simulink model "MODELO_CORRECTO_BERGMAN_BASE"  (R2019b)
settings: Solver=VariableStepAuto  StartTime=0.0  StopTime=50000  RelTol=1e-3
undefined symbols (not defined in the file): Gb, Ib, n, p1, p2, p3, p5, p6
libraries: simulink x29
settings Model: Creator=USUARIO  LastModifiedBy=USUARIO

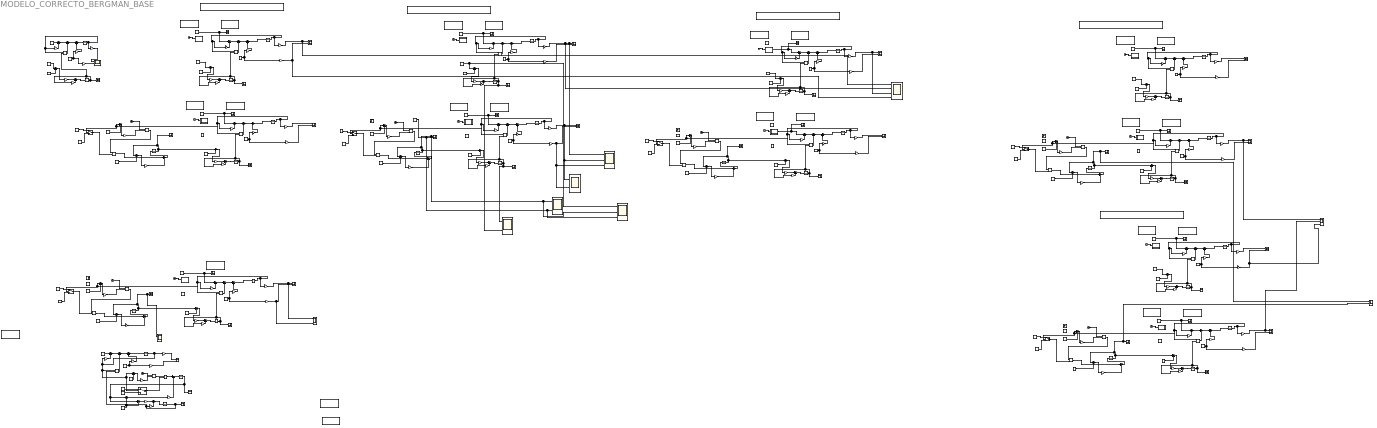
== system MODELO_CORRECTO_BERGMAN_BASE ==
  "    " : Gain  Gain=p6
  Clock{,1..17} (18 alike) : Clock
  Constant{1..11} (11 alike) : Constant  Value=0
  Factor conversión : Gain  Gain=18
  "Factor conversión    " : Gain  Gain=18
  Factor de conversión : Gain  Gain=18
  "Factor de conversión " : Gain  Gain=18
  False : Constant
  Gain{1,5,8,10,13..14,20,23,25..26,32,35,37..38,44,47,49..50,56,59,61,65,67,69,71,75} (26 alike) : Gain  Gain=p1
  Gain{2,11,15,17,27,29,39,41,51,53,62,68,70} (13 alike) : Gain  Gain=p3
  Gain{3..4,7,12,16,18..19,22,28,30..31,34,40,42..43,46,52,54..55,58,63..64} (22 alike) : Gain  Gain=18
  Gain{6,9,21,24,33,36,45,48,57,60,66,72,76} (13 alike) : Gain  Gain=p2
  "Glucosa " : Constant  Value=12
  Glucosa {2..5} (4 alike) : Constant  Value=7
  Glucosa basal : Constant  Value=Gb
  "Glucosa basal         " : Constant  Value=Gb
  Glucosa basal{1..4,9..10,13,17..18,21} (10 alike) : Constant  Value=4.5
  Glucosa basal{5,7,11,15,19,22} (6 alike) : Constant
  Glucosa basal{6,8,12,16,20,23} (6 alike) : Constant  Value=0
  Glucosa basal14 : Constant  Value=5.11
  Grafica ingesta D{1..10,12} (11 alike) : Scope
  Grafica ingesta D11 : Scope  NumInputPorts=2
  Gráfica de la glucosa : Scope  NumInputPorts=2
  Gráfica glucosa : Scope  NumInputPorts=2
  Gráfica insulina activa : Scope
  "Gráfica insulina activa       " : Scope
  Gráfica insulina variable : Scope
  INSULINA : Scope  NumInputPorts=2
  INSULINA{1..5} (5 alike) : Scope
  INSULINA7 : Scope  NumInputPorts=2
  Ib{,1..2,4..5} (5 alike) : Constant  Value=12
  Ib3 : Constant  Value=11
  Ingesta : Constant  Value=0
  "Ingesta      " : Constant  Value=0
  Ingesta 75 g1 : MATLAB Function  TreatAsAtomicUnit=on
  Ingesta 75 g10 : MATLAB Function  TreatAsAtomicUnit=on
  Ingesta 75 g11 : MATLAB Function  TreatAsAtomicUnit=on
  Ingesta 75 g2 : MATLAB Function  TreatAsAtomicUnit=on
  Ingesta 75 g3 : MATLAB Function  TreatAsAtomicUnit=on
  Ingesta 75 g4 : MATLAB Function  TreatAsAtomicUnit=on
  Ingesta 75 g5 : MATLAB Function  TreatAsAtomicUnit=on
  Ingesta 75 g6 : MATLAB Function  TreatAsAtomicUnit=on
  Ingesta 75 g7 : MATLAB Function  TreatAsAtomicUnit=on
  Ingesta 75 g8 : MATLAB Function  TreatAsAtomicUnit=on
  Ingesta 75 g9 : MATLAB Function  TreatAsAtomicUnit=on
  "Insulina basal     " : Constant  Value=Ib
  Insulina basal{1..6,8..11} (10 alike) : Constant  Value=12
  Insulina basal7 : Constant  Value=11
  Insulina constante : Constant  Value=Ib
  Integrator{1,5,16,19,21,24} (6 alike) : Integrator  InitialCondition=7.5
  Integrator{3,8,10,13,32} (5 alike) : Integrator  InitialCondition=4.5
  Integrator{4,11,14,17,22,27,30} (7 alike) : Integrator  InitialCondition=12
  Integrator{2,6..7,9,12,15,18,20,23,25,28,31,33} (13 alike) : Integrator
  Integrator26 : Integrator  InitialCondition=8
  Integrator29 : Integrator  InitialCondition=8
  Model Info1 : simulink/Model-Wide Utilities/Model Info  Frame=on  DisplayStringWithTags=|  HorizontalTextAlignment=Center  LeftAlignmentValue=0.5
      | Insulina constante 
      | igual a la basal
      | 
      | I(0) = Ib
  Model Info10 : simulink/Model-Wide Utilities/Model Info  Frame=on  DisplayStringWithTags=|  HorizontalTextAlignment=Center  LeftAlignmentValue=0.5
      | MODELO ORIGINAL
      | 
      | 
      | PERSONA NO DIABETICA
      | 
      | CON INSULINA CONSTANTE
  Model Info11 : simulink/Model-Wide Utilities/Model Info  Frame=on  DisplayStringWithTags=|  HorizontalTextAlignment=Center  LeftAlignmentValue=0.5
      | Insulina constante 
      | igual a la basal
      | 
      | I(0) = Ib
  Model Info12 : simulink/Model-Wide Utilities/Model Info  Frame=on  DisplayStringWithTags=|  HorizontalTextAlignment=Center  LeftAlignmentValue=0.5
      | MODELO ORIGINAL
      | 
      | 
      | PERSONA NO DIABETICA
      | 
      | CON INSULINA VARIABLE
  Model Info13 : simulink/Model-Wide Utilities/Model Info  Frame=on  DisplayStringWithTags=TRAS INGESTA  HorizontalTextAlignment=Center  LeftAlignmentValue=0.5
  Model Info14 : simulink/Model-Wide Utilities/Model Info  Frame=on  DisplayStringWithTags=AYUNAS  HorizontalTextAlignment=Center  LeftAlignmentValue=0.5
  Model Info15 : simulink/Model-Wide Utilities/Model Info  Frame=on  DisplayStringWithTags=INGESTA  HorizontalTextAlignment=Center  LeftAlignmentValue=0.5
  Model Info16 : simulink/Model-Wide Utilities/Model Info  Frame=on  DisplayStringWithTags=|  HorizontalTextAlignment=Center  LeftAlignmentValue=0.5
      | Insulina constante 
      | igual a la basal
      | 
      | I(0) = Ib
  Model Info17 : simulink/Model-Wide Utilities/Model Info  Frame=on  DisplayStringWithTags=|  HorizontalTextAlignment=Center  LeftAlignmentValue=0.5
      | TRAS INGESTA
      | 
      | PACIENTE 2:
      | IB=11
      | GB=5.11
  Model Info18 : simulink/Model-Wide Utilities/Model Info  Frame=on  DisplayStringWithTags=|  HorizontalTextAlignment=Center  LeftAlignmentValue=0.5
      | MODELO ORIGINAL
      | 
      | 
      | PERSONA NO DIABETICA
      | 
      | CON INSULINA CONSTANTE
  Model Info19 : simulink/Model-Wide Utilities/Model Info  Frame=on  DisplayStringWithTags=|  HorizontalTextAlignment=Center  LeftAlignmentValue=0.5
      | Insulina constante 
      | igual a la basal
      | 
      | I(0) = Ib
  Model Info2 : simulink/Model-Wide Utilities/Model Info  Frame=on  DisplayStringWithTags=|  HorizontalTextAlignment=Center  LeftAlignmentValue=0.5
      | MODELO ORIGINAL
      | 
      | 
      | PERSONA NO DIABETICA
      | 
      | CON INSULINA CONSTANTE
  Model Info20 : simulink/Model-Wide Utilities/Model Info  Frame=on  DisplayStringWithTags=|  HorizontalTextAlignment=Center  LeftAlignmentValue=0.5
      | MODELO ORIGINAL
      | 
      | 
      | PERSONA NO DIABETICA
      | 
      | CON INSULINA VARIABLE
  Model Info21 : simulink/Model-Wide Utilities/Model Info  Frame=on  DisplayStringWithTags=|  HorizontalTextAlignment=Center  LeftAlignmentValue=0.5
      | Insulina constante 
      | igual a la basal
      | 
      | I(0) = Ib
  Model Info22 : simulink/Model-Wide Utilities/Model Info  Frame=on  DisplayStringWithTags=|  HorizontalTextAlignment=Center  LeftAlignmentValue=0.5
      | TRAS INGESTA
      | 
      | PACIENTE 2:
      | IB=11
      | GB=5.11
  Model Info23 : simulink/Model-Wide Utilities/Model Info  Frame=on  DisplayStringWithTags=|  HorizontalTextAlignment=Center  LeftAlignmentValue=0.5
      | MODELO ORIGINAL
      | 
      | 
      | PERSONA NO DIABETICA
      | 
      | CON INSULINA CONSTANTE
  Model Info24 : simulink/Model-Wide Utilities/Model Info  Frame=on  DisplayStringWithTags=|  HorizontalTextAlignment=Center  LeftAlignmentValue=0.5
      | Insulina constante 
      | igual a la basal
      | 
      | I(0) = Ib
  Model Info25 : simulink/Model-Wide Utilities/Model Info  Frame=on  DisplayStringWithTags=|  HorizontalTextAlignment=Center  LeftAlignmentValue=0.5
      | MODELO ORIGINAL
      | 
      | 
      | PERSONA NO DIABETICA
      | 
      | CON INSULINA VARIABLE
  Model Info26 : simulink/Model-Wide Utilities/Model Info  Frame=on  DisplayStringWithTags=|  HorizontalTextAlignment=Center  LeftAlignmentValue=0.5
      | Insulina constante 
      | igual a la basal
      | 
      | I(0) = Ib
  Model Info27 : simulink/Model-Wide Utilities/Model Info  Frame=on  DisplayStringWithTags=ejemplo para p5  HorizontalTextAlignment=Center  LeftAlignmentValue=0.5
  Model Info28 : simulink/Model-Wide Utilities/Model Info  Frame=on  DisplayStringWithTags=|  HorizontalTextAlignment=Center  LeftAlignmentValue=0.5
      | Insulina constante 
      | igual a la basal
      | 
      | I(0) = Ib
  Model Info29 : simulink/Model-Wide Utilities/Model Info  Frame=on  DisplayStringWithTags=|  HorizontalTextAlignment=Center  LeftAlignmentValue=0.5
      | MODELO ORIGINAL
      | 
      | 
      | PERSONA NO DIABETICA
      | 
      | CON INSULINA VARIABLE
  Model Info3 : simulink/Model-Wide Utilities/Model Info  Frame=on  DisplayStringWithTags=|  HorizontalTextAlignment=Center  LeftAlignmentValue=0.5
      | Insulina constante 
      | igual a la basal
      | 
      | I(0) = Ib
  Model Info4 : simulink/Model-Wide Utilities/Model Info  Frame=on  DisplayStringWithTags=|  HorizontalTextAlignment=Center  LeftAlignmentValue=0.5
      | MODELO ORIGINAL
      | 
      | 
      | PERSONA NO DIABETICA
      | 
      | CON INSULINA VARIABLE
  Model Info5 : simulink/Model-Wide Utilities/Model Info  Frame=on  DisplayStringWithTags=|  HorizontalTextAlignment=Center  LeftAlignmentValue=0.5
      | Insulina constante 
      | igual a la basal
      | 
      | I(0) = Ib
  Model Info6 : simulink/Model-Wide Utilities/Model Info  Frame=on  DisplayStringWithTags=|  HorizontalTextAlignment=Center  LeftAlignmentValue=0.5
      | MODELO ORIGINAL
      | 
      | 
      | PERSONA NO DIABETICA
      | 
      | CON INSULINA CONSTANTE
  Model Info7 : simulink/Model-Wide Utilities/Model Info  Frame=on  DisplayStringWithTags=|  HorizontalTextAlignment=Center  LeftAlignmentValue=0.5
      | Insulina constante 
      | igual a la basal
      | 
      | I(0) = Ib
  Model Info8 : simulink/Model-Wide Utilities/Model Info  Frame=on  DisplayStringWithTags=|  HorizontalTextAlignment=Center  LeftAlignmentValue=0.5
      | MODELO ORIGINAL
      | 
      | 
      | PERSONA NO DIABETICA
      | 
      | CON INSULINA VARIABLE
  Model Info9 : simulink/Model-Wide Utilities/Model Info  Frame=on  DisplayStringWithTags=|  HorizontalTextAlignment=Center  LeftAlignmentValue=0.5
      | Insulina constante 
      | igual a la basal
      | 
      | I(0) = Ib
  Product{1..27} (27 alike) : Product
  Scope : Scope  NumInputPorts=2
  Scope1 : Scope  NumInputPorts=2
  Scope2 : Scope  NumInputPorts=2
  Scope3 : Scope  NumInputPorts=3
  Scope4 : Scope  NumInputPorts=4
  Step{,2..5} (5 alike) : Step  Time=10  Before=7  After=4  SampleTime=0
  Sum{1..2,4..11,13,15..16,18..23,25..26,28..42,44..45,47..55,57..58,60..66,68..74,76..81,83..86} (73 alike) : Sum  Inputs=|+-
  Sum{3,12,14,17,24,27,43,46,56,59,67,75,82} (13 alike) : Sum  Inputs=|++
  Switch{,1..5} (6 alike) : Switch  Criteria=u2 > Threshold  Threshold=5
  Switch: Páncreas : Switch  Criteria=u2 > Threshold  Threshold=p5
  True : Constant  Value=0
  glucosa con y sin insulina variable : Scope  NumInputPorts=3
  i(T){,1..10} (11 alike) : Constant  Value=12
  insulina activa{1..11} (11 alike) : Scope
  insulina basal : Constant  Value=Ib
  mODELO ORIGINAL{,1..9,11} (11 alike) : Scope  NumInputPorts=2
  mODELO ORIGINAL10 : Scope  NumInputPorts=3
  mODELO ORIGINAL13 : Scope  NumInputPorts=3
  p{1,3,5,7,9,11} (6 alike) : Constant  Value=5
  p{2,4,6,8,10,12} (6 alike) : Gain  Gain=p6
  p4 = n{,1..5} (6 alike) : Gain  Gain=n
  "p4 = n    " : Gain  Gain=n
  "p5   " : Constant  Value=p5
  wires:
  Sum31/1 -> p6/1
  Product8/1 -> Sum33/1
  Glucosa basal7/1 -> Switch/1  "glucosa basal"
  Sum33/1 -> Integrator14/1
  p6/1 -> Product7/2
  Clock/1 -> Product7/1
  p4 = n/1 -> Sum33/2
  Ib/1 -> Sum32/2  "glucosa basal"
  Sum32/1 -> p4 = n/1
  Glucosa basal8/1 -> Switch/3  "glucosa basal"
  Switch/1 -> Product8/2
  Integrator14/1 -> Sum1/1, Scope3/2, Scope1/1, INSULINA/1, Sum32/1  "Insulina con insulina variable"
  p5/1 -> Sum31/2  "glucosa basal"
  Product7/1 -> Product8/1
  Integrator5/1 -> Gain12/1, Product3/1, Gain10/1  "G(t)"
  Gain12/1 -> Scope4/2, glucosa con y sin insulina variable/1, mODELO ORIGINAL/1  "Glucosa con insulina cte"
  Constant4/1 -> Grafica ingesta D2/1, Sum11/1
  i(T)/1 -> Scope3/1, Sum10/1  "Insulina con insulina cte"
  Gain10/1 -> Sum11/2
  Insulina basal3/1 -> Sum10/2  "insulina basal"
  Sum10/1 -> Gain11/1
  Gain11/1 -> Sum13/1
  Sum8/1 -> Sum12/1
  Gain9/1 -> Sum13/2
  Sum12/1 -> Integrator5/1
  Glucosa basal2/1 -> Gain8/1, Gain7/1  "glucosa basal"
  Product3/1 -> Sum8/2
  Clock2/1 -> Ingesta 75 g2/1(in)
  Sum13/1 -> Integrator6/1
  Integrator6/1 -> insulina activa2/1, Scope2/2, Product3/2, Gain9/1  "Insulina activa con insulina cte"
  Gain8/1 -> Sum12/2
  Sum11/1 -> Sum8/1
  Gain7/1 -> mODELO ORIGINAL/2  "glucosa basal"
  Integrator1/1 -> Gain3/1, Sum31/1, Switch/2, Product1/1, Gain1/1  "G(t)"
  Gain3/1 -> glucosa con y sin insulina variable/2, Scope/1, mODELO ORIGINAL1/1  "Glucosa con insulina variable"
  Sum3/1 -> Integrator1/1
  Constant1/1 -> Grafica ingesta D1/1, Sum2/1
  Sum4/1 -> Integrator2/1
  Product1/1 -> Sum5/2
  Sum2/1 -> Sum5/1
  Gain5/1 -> Sum3/2
  Gain4/1 -> Scope/2, glucosa con y sin insulina variable/3, mODELO ORIGINAL1/2  "Glucosa basal"
  Integrator2/1 -> insulina activa1/1, Scope2/1, Product1/2, Gain6/1  "Insulina activa con insulina variable"
  Glucosa basal1/1 -> Gain5/1, Gain4/1  "glucosa basal"
  Gain6/1 -> Sum4/2
  Insulina basal1/1 -> Sum1/2  "insulina basal"
  Clock1/1 -> Ingesta 75 g1/1(in)
  Gain2/1 -> Sum4/1
  Sum1/1 -> Gain2/1
  Gain1/1 -> Sum2/2
  Sum5/1 -> Sum3/1
  Gain18/1 -> mODELO ORIGINAL3/1  "Glucosa tras ingesta con insulina modelada"
  Integrator3/1 -> Gain18/1, Sum18/1, Switch1/2, Product2/1, Gain13/1  "G(t)"
  Glucosa basal3/1 -> Gain20/1, Gain19/1  "glucosa basal"
  Integrator7/1 -> insulina activa3/1, Product2/2, Gain21/1  "X(t)"
  Integrator8/1 -> Gain16/1, Product4/1, Gain14/1  "G(t)"
  Sum16/1 -> Sum22/1
  Sum21/1 -> Integrator7/1
  Constant2/1 -> Grafica ingesta D3/1, Sum16/1
  Gain16/1 -> Scope4/1, mODELO ORIGINAL2/1  "Ayunas"
  Product5/1 -> Product6/1
  p1/1 -> Sum18/2  "glucosa basal"
  Integrator4/1 -> Sum6/1, INSULINA1/1, Sum19/1  "I(t)"
  Glucosa basal6/1 -> Switch1/3  "glucosa basal"
  Sum19/1 -> p4 = n1/1
  Sum17/1 -> Integrator3/1
  Clock3/1 -> Product5/1
  p2/1 -> Product5/2
  Product6/1 -> Sum20/1
  Gain20/1 -> Sum17/2
  Sum18/1 -> p2/1
  Constant3/1 -> Grafica ingesta D4/1, Sum9/1
  Sum6/1 -> Gain17/1
  Gain17/1 -> Sum21/1
  Sum14/1 -> Integrator8/1
  Clock4/1 -> Ingesta 75 g3/1(in)
  Insulina basal2/1 -> Sum6/2  "insulina basal"
  Product4/1 -> Sum23/2
  Sum9/1 -> Sum23/1
  Switch1/1 -> Product6/2
  Gain23/1 -> Sum14/2
  Gain22/1 -> Scope4/4, mODELO ORIGINAL2/2  "Glucosa basal"
  Integrator9/1 -> insulina activa4/1, Product4/2, Gain24/1  "X(t)"
  Sum22/1 -> Sum17/1
  Gain14/1 -> Sum9/2
  Gain21/1 -> Sum21/2
  Sum23/1 -> Sum14/1
  Glucosa basal4/1 -> Gain23/1, Gain22/1  "glucosa basal"
  Sum20/1 -> Integrator4/1
  Product2/1 -> Sum22/2
  i(T)2/1 -> Sum7/1
  Gain24/1 -> Sum15/2
  Gain15/1 -> Sum15/1
  Gain19/1 -> mODELO ORIGINAL3/2  "glucosa basal"
  Ib1/1 -> Sum19/2  "glucosa basal"
  Sum7/1 -> Gain15/1
  Glucosa basal5/1 -> Switch1/1  "glucosa basal"
  Insulina basal4/1 -> Sum7/2  "insulina basal"
  Clock5/1 -> Ingesta 75 g4/1(in)
  p4 = n1/1 -> Sum20/2
  Gain13/1 -> Sum16/2
  Sum15/1 -> Integrator9/1
  Integrator12/1 -> insulina activa5/1, Product9/2, Gain33/1  "X(t)"
  Integrator13/1 -> Gain28/1, Product10/1, Gain26/1  "G(t)"
  Sum26/1 -> Sum35/1
  Glucosa basal9/1 -> Gain32/1, Gain31/1  "glucosa basal"
  Integrator10/1 -> Gain30/1, Sum28/1, Switch2/2, Product9/1, Gain25/1  "G(t)"
  Gain30/1 -> mODELO ORIGINAL5/1  "Glucosa ingesta con insulina modelada"
  Clock8/1 -> Ingesta 75 g6/1(in)
  Insulina basal6/1 -> Sum38/2  "insulina basal"
  Sum38/1 -> Gain27/1
  Glucosa basal11/1 -> Switch2/1  "glucosa basal"
  Ib2/1 -> Sum29/2  "glucosa basal"
  Gain25/1 -> Sum26/2
  Product9/1 -> Sum35/2
  Sum30/1 -> Integrator11/1
  i(T)4/1 -> Sum38/1
  Gain36/1 -> Sum25/2
  Gain31/1 -> mODELO ORIGINAL5/2  "glucosa basal"
  p4 = n2/1 -> Sum30/2
  Glucosa basal10/1 -> Gain35/1, Gain34/1  "glucosa basal"
  Gain27/1 -> Sum25/1
  Gain33/1 -> Sum34/2
  Gain26/1 -> Sum39/2
  Integrator15/1 -> insulina activa6/1, Product10/2, Gain36/1  "X(t)"
  Gain35/1 -> Sum24/2
  Sum35/1 -> Sum27/1
  Clock7/1 -> Ingesta 75 g5/1(in)
  Sum39/1 -> Sum36/1
  Switch2/1 -> Product12/2
  Gain34/1 -> mODELO ORIGINAL4/2  "glucosa basal"
  Insulina basal5/1 -> Sum37/2  "insulina basal"
  Product10/1 -> Sum36/2
  Gain32/1 -> Sum27/2
  Sum24/1 -> Integrator13/1
  Sum28/1 -> p4/1
  Sum37/1 -> Gain29/1
  Gain29/1 -> Sum34/1
  Product12/1 -> Sum30/1
  Sum29/1 -> p4 = n2/1
  p4/1 -> Product11/2
  Glucosa basal12/1 -> Switch2/3  "glucosa basal"
  Sum27/1 -> Integrator10/1
  Integrator11/1 -> Sum37/1, INSULINA2/1, Sum29/1  "I(t)"
  Sum36/1 -> Sum24/1
  Clock6/1 -> Product11/1
  Product11/1 -> Product12/1
  Sum34/1 -> Integrator12/1
  p3/1 -> Sum28/2  "p5"
  Sum25/1 -> Integrator15/1
  Gain28/1 -> Scope4/3, mODELO ORIGINAL4/1  "Ingesta"
  Ingesta 75 g6/1(D) -> Grafica ingesta D6/1, Sum39/1
  Ingesta 75 g5/1(D) -> Grafica ingesta D5/1, Sum26/1
  Gain42/1 -> mODELO ORIGINAL10/1, mODELO ORIGINAL7/1  "Glucosa tras ingesta PACIENTE 2"
  Integrator16/1 -> Gain42/1, Sum47/1, Switch3/2, Product13/1, Gain37/1  "G(t)"
  Glucosa basal13/1 -> Gain44/1, Gain43/1  "glucosa basal"
  Integrator18/1 -> insulina activa7/1, Product13/2, Gain45/1  "X(t)"
  Integrator19/1 -> Gain40/1, Product14/1, Gain38/1  "G(t)"
  Sum45/1 -> Sum51/1
  Sum50/1 -> Integrator18/1
  Constant7/1 -> Grafica ingesta D7/1, Sum45/1
  Gain40/1 -> mODELO ORIGINAL6/1  "Glucosa tras ingesta con insulina constante"
  Product15/1 -> Product16/1
  p7/1 -> Sum47/2  "glucosa basal"
  Integrator17/1 -> Sum40/1, Grafica ingesta D11/1, INSULINA3/1, Sum48/1  "I(t) PACIENTE 2"
  Glucosa basal16/1 -> Switch3/3  "glucosa basal"
  Sum48/1 -> p4 = n3/1
  Sum46/1 -> Integrator16/1
  Clock9/1 -> Product15/1
  p8/1 -> Product15/2
  Product16/1 -> Sum49/1
  Gain44/1 -> Sum46/2
  Sum47/1 -> p8/1
  Constant8/1 -> Grafica ingesta D8/1, Sum42/1
  Sum40/1 -> Gain41/1
  Gain41/1 -> Sum50/1
  Sum43/1 -> Integrator19/1
  Clock10/1 -> Ingesta 75 g7/1(in)
  Insulina basal7/1 -> Sum40/2  "insulina basal"
  Product14/1 -> Sum52/2
  Sum42/1 -> Sum52/1
  Switch3/1 -> Product16/2
  Gain47/1 -> Sum43/2
  Gain46/1 -> mODELO ORIGINAL6/2  "glucosa basal"
  Integrator20/1 -> insulina activa8/1, Product14/2, Gain48/1  "X(t)"
  Sum51/1 -> Sum46/1
  Gain38/1 -> Sum42/2
  Gain45/1 -> Sum50/2
  Sum52/1 -> Sum43/1
  Glucosa basal14/1 -> Gain47/1, Gain46/1  "glucosa basal"
  Sum49/1 -> Integrator17/1
  Product13/1 -> Sum51/2
  i(T)6/1 -> Sum41/1
  Gain48/1 -> Sum44/2
  Gain39/1 -> Sum44/1
  Gain43/1 -> mODELO ORIGINAL7/2  "glucosa basal"
  Ib3/1 -> Sum48/2  "glucosa basal"
  Sum41/1 -> Gain39/1
  Glucosa basal15/1 -> Switch3/1  "glucosa basal"
  Insulina basal8/1 -> Sum41/2  "insulina basal"
  Clock11/1 -> Ingesta 75 g8/1(in)
  p4 = n3/1 -> Sum49/2
  Gain37/1 -> Sum45/2
  Sum44/1 -> Integrator20/1
  Glucosa basal17/1 -> Gain56/1, Gain55/1  "glucosa basal"
  Integrator21/1 -> Gain54/1, Sum60/1, Switch4/2, Product17/1, Gain49/1  "G(t)"
  Sum64/1 -> Sum59/1
  Sum65/1 -> Sum56/1
  Gain57/1 -> Sum63/2
  Gain59/1 -> Sum56/2
  Sum55/1 -> Sum65/1
  Sum56/1 -> Integrator24/1
  Constant10/1 -> Grafica ingesta D10/1, Sum55/1
  Clock12/1 -> Ingesta 75 g9/1(in)
  p10/1 -> Product19/2
  Product20/1 -> Sum62/1
  Gain53/1 -> Sum63/1
  Glucosa basal20/1 -> Switch4/3  "glucosa basal"
  Sum59/1 -> Integrator21/1
  Sum61/1 -> p4 = n4/1
  Gain50/1 -> Sum55/2
  Integrator22/1 -> Sum53/1, Grafica ingesta D11/2, INSULINA4/1, Sum61/1  "I(t) PACIENTE 1"
  Integrator25/1 -> insulina activa10/1, Product18/2, Gain60/1  "X(t)"
  Gain52/1 -> mODELO ORIGINAL8/1  "Glucosa tras ingesta con insulina constante"
  Clock14/1 -> Product19/1
  Gain56/1 -> Sum59/2
  p9/1 -> Sum60/2  "glucosa basal"
  Product19/1 -> Product20/1
  Constant9/1 -> Grafica ingesta D9/1, Sum58/1
  Sum63/1 -> Integrator23/1
  Sum60/1 -> p10/1
  Product18/1 -> Sum65/2
  Sum53/1 -> Gain53/1
  Integrator23/1 -> insulina activa9/1, Product17/2, Gain57/1  "X(t)"
  Integrator24/1 -> Gain52/1, Product18/1, Gain50/1  "G(t)"
  p4 = n4/1 -> Sum62/2
  Clock13/1 -> Ingesta 75 g10/1(in)
  Sum58/1 -> Sum64/1
  Sum57/1 -> Integrator25/1
  Gain49/1 -> Sum58/2
  Switch4/1 -> Product20/2
  Gain60/1 -> Sum57/2
  Gain51/1 -> Sum57/1
  Insulina basal9/1 -> Sum53/2  "insulina basal"
  Ib4/1 -> Sum61/2  "glucosa basal"
  Insulina basal10/1 -> Sum54/2  "insulina basal"
  Glucosa basal19/1 -> Switch4/1  "glucosa basal"
  Product17/1 -> Sum64/2
  Glucosa basal18/1 -> Gain59/1, Gain58/1  "glucosa basal"
  i(T)8/1 -> Sum54/1
  Gain58/1 -> mODELO ORIGINAL8/2, mODELO ORIGINAL10/3  "glucosa basal"
  Gain54/1 -> mODELO ORIGINAL10/2, mODELO ORIGINAL9/1  "Glucosa tras ingesta PACIENTE 1"
  Sum62/1 -> Integrator22/1
  Gain55/1 -> mODELO ORIGINAL9/2  "glucosa basal"
  Sum54/1 -> Gain51/1
  "Glucosa "/1 -> Scope3/3, Scope1/2, INSULINA/2  "Insulina Basal"
  Sum72/1 -> Sum67/1
  p4 = n5/1 -> Sum70/2
  Product23/1 -> Sum70/1
  Integrator28/1 -> insulina activa11/1, Product21/2, Gain66/1  "X(t)"
  Gain65/1 -> Sum67/2
  Sum71/1 -> Integrator28/1
  Gain62/1 -> Sum71/1
  Ib5/1 -> Sum69/2  "glucosa basal"
  Sum68/1 -> p12/1
  p11/1 -> Sum68/2  "glucosa basal"
  Sum70/1 -> Integrator27/1
  Gain61/1 -> Sum66/2
  Clock16/1 -> Ingesta 75 g11/1(in)
  Constant11/1 -> Grafica ingesta D12/1, Sum66/1
  Integrator26/1 -> Gain63/1, Sum68/1, Switch5/2, Product21/1, Gain61/1  "G(t)"
  Sum66/1 -> Sum72/1
  Switch5/1 -> Product23/2
  Insulina basal11/1 -> Sum73/2  "insulina basal"
  Sum73/1 -> Gain62/1
  Product22/1 -> Product23/1
  Glucosa basal23/1 -> Switch5/3  "glucosa basal"
  p12/1 -> Product22/2
  Clock15/1 -> Product22/1
  Sum67/1 -> Integrator26/1
  Sum69/1 -> p4 = n5/1
  Gain63/1 -> mODELO ORIGINAL13/1, mODELO ORIGINAL11/1  "p5 = 90 mg/dL"
  Integrator27/1 -> Sum73/1, INSULINA7/1, INSULINA5/1, Sum69/1  "I(t)"
  Gain66/1 -> Sum71/2
  Glucosa basal22/1 -> Switch5/1  "glucosa basal"
  Product21/1 -> Sum72/2
  Glucosa basal21/1 -> Gain65/1, Gain64/1  "glucosa basal"
  Gain64/1 -> mODELO ORIGINAL13/3, mODELO ORIGINAL11/2  "glucosa basal"
  Glucosa basal/1 -> Factor conversión/1, Gain71/1
  Factor conversión/1 -> Gráfica glucosa/2  "Glucosa basal"
  Sum75/1 -> Integrator29/1
  Integrator30/1 -> Gráfica insulina variable/1, Sum81/1, Sum77/1
  Sum77/1 -> "p4 = n    "/1
  Sum81/1 -> Gain68/1
  True/1 -> Switch: Páncreas/3
  Product25/1 -> Product26/1
  Sum74/1 -> Sum80/1
  Ingesta/1 -> Sum74/1
  Switch: Páncreas/1 -> Product26/2
  Product24/1 -> Sum80/2
  "p5   "/1 -> Sum76/2
  Gain72/1 -> Sum79/2
  Sum76/1 -> "    "/1
  Clock17/1 -> Product25/1
  Gain68/1 -> Sum79/1
  Integrator29/1 -> Sum76/1, Switch: Páncreas/2, Product24/1, Gain67/1, "Factor conversión    "/1  "G(t)"
  Gain67/1 -> Sum74/2
  insulina basal/1 -> Sum77/2, Sum81/2
  Sum78/1 -> Integrator30/1
  "    "/1 -> Product25/2
  "Factor conversión    "/1 -> Gráfica glucosa/1  "G(t)"
  "p4 = n    "/1 -> Sum78/2
  Gain71/1 -> Sum75/2
  False/1 -> Switch: Páncreas/1
  Product26/1 -> Sum78/1
  Sum79/1 -> Integrator31/1
  Sum80/1 -> Sum75/1
  Integrator31/1 -> Gráfica insulina activa/1, Gain72/1, Product24/2  "X(t)"
  Sum82/1 -> Integrator32/1
  Sum85/1 -> Gain70/1
  "Insulina basal     "/1 -> Sum85/2
  Sum86/1 -> Sum84/1
  Factor de conversión/1 -> Gráfica de la glucosa/2  "Glucosa basal"
  Integrator33/1 -> "Gráfica insulina activa       "/1, Product27/2, Gain76/1  "X(t)"
  "Glucosa basal         "/1 -> Gain75/1, Factor de conversión/1
  Sum83/1 -> Integrator33/1
  Integrator32/1 -> Product27/1, Gain69/1, "Factor de conversión "/1  "G(t)"
  Sum84/1 -> Sum82/1
  Product27/1 -> Sum84/2
  Gain70/1 -> Sum83/1
  Gain69/1 -> Sum86/2
  "Ingesta      "/1 -> Sum86/1
  Insulina constante/1 -> Sum85/1
  Gain75/1 -> Sum82/2
  Gain76/1 -> Sum83/2
  "Factor de conversión "/1 -> Gráfica de la glucosa/1  "G(t)"

== matlab function MODELO_CORRECTO_BERGMAN_BASE/Ingesta 75 g1 ==
  data: in input; D output
function D = comida(in)
% Variables de entrada en la funcion
t = in(1) %- 8*60*60; % Ajuste para iniciar a las 8 de la mañana
 
% Parámetros del modelo
Ag = 0.8; % adimensional
Tmaxi = 55*60; % s
Vg = 13.79; % L
Tmaxg = 40*60; % s
t1 = 0;
Dg = 0;
f = 1000/180; % factor de conversión de g a mmol
 
% Comidas (perturbaciones) a lo largo de un día
if t >= 0 && t < 180*60 % ingesta de 75 g de HC
    t1 = 0;
    Dg = 50*f;
end
 
% Ecuación
D = (Dg*Ag*(t-t1)*exp(-(t-t1)/Tmaxi))/(Vg*Tmaxg^2);

== matlab function MODELO_CORRECTO_BERGMAN_BASE/Ingesta 75 g2 ==
  data: in input; D output
function D = comida(in)
% Variables de entrada en la funcion
t = in(1) %- 8*60*60; % Ajuste para iniciar a las 8 de la mañana
 
% Parámetros del modelo
Ag = 0.8; % adimensional
Tmaxi = 55*60; % s
Vg = 13.79; % L
Tmaxg = 40*60; % s
t1 = 0;
Dg = 0;
f = 1000/180; % factor de conversión de g a mmol
 
% Comidas (perturbaciones) a lo largo de un día
if t >= 0 && t < 180*60 % ingesta de 75 g de HC
    t1 = 0;
    Dg = 50*f;
end
 
% Ecuación
D = (Dg*Ag*(t-t1)*exp(-(t-t1)/Tmaxi))/(Vg*Tmaxg^2);

== matlab function MODELO_CORRECTO_BERGMAN_BASE/Ingesta 75 g3 ==
  data: in input; D output
function D = comida(in)
% Variables de entrada en la funcion
t = in(1) %- 8*60*60; % Ajuste para iniciar a las 8 de la mañana
 
% Parámetros del modelo
Ag = 0.8; % adimensional
Tmaxi = 55*60; % s
Vg = 13.79; % L
Tmaxg = 40*60; % s
t1 = 0;
Dg = 0;
f = 1000/180; % factor de conversión de g a mmol
 
% Comidas (perturbaciones) a lo largo de un día
if t >= 0 && t < 180*60 % ingesta de 75 g de HC
    t1 = 0;
    Dg = 50*f;
end
 
% Ecuación
D = (Dg*Ag*(t-t1)*exp(-(t-t1)/Tmaxi))/(Vg*Tmaxg^2);

== matlab function MODELO_CORRECTO_BERGMAN_BASE/Ingesta 75 g4 ==
  data: in input; D output
function D = comida(in)
% Variables de entrada en la funcion
t = in(1) %- 8*60*60; % Ajuste para iniciar a las 8 de la mañana
 
% Parámetros del modelo
Ag = 0.8; % adimensional
Tmaxi = 55*60; % s
Vg = 13.79; % L
Tmaxg = 40*60; % s
t1 = 0;
Dg = 0;
f = 1000/180; % factor de conversión de g a mmol
 
% Comidas (perturbaciones) a lo largo de un día
if t >= 0 && t < 180*60 % ingesta de 75 g de HC
    t1 = 0;
    Dg = 50*f;
end
 
% Ecuación
D = (Dg*Ag*(t-t1)*exp(-(t-t1)/Tmaxi))/(Vg*Tmaxg^2);

== matlab function MODELO_CORRECTO_BERGMAN_BASE/Ingesta 75 g5 ==
  data: in input; D output
function D = comida(in)
% Variables de entrada en la funcion
t = in(1) %- 8*60*60; % Ajuste para iniciar a las 8 de la mañana
 
% Parámetros del modelo
Ag = 0.8; % adimensional
Tmaxi = 55*60; % s
Vg = 13.79; % L
Tmaxg = 40*60; % s
t1 = 0;
Dg = 0;
f = 1000/180; % factor de conversión de g a mmol
 
% Comidas (perturbaciones) a lo largo de un día
if t >= 0 && t < 180*60 % ingesta de 75 g de HC
    t1 = 0;
    Dg = 50*f;
end
 
% Ecuación
D = (Dg*Ag*(t-t1)*exp(-(t-t1)/Tmaxi))/(Vg*Tmaxg^2);

== matlab function MODELO_CORRECTO_BERGMAN_BASE/Ingesta 75 g6 ==
  data: in input; D output
function D = comida(in)
% Variables de entrada en la funcion
t = in(1) %- 8*60*60; % Ajuste para iniciar a las 8 de la mañana
 
% Parámetros del modelo
Ag = 0.8; % adimensional
Tmaxi = 55*60; % s
Vg = 13.79; % L
Tmaxg = 40*60; % s
t1 = 0;
Dg = 0;
f = 1000/180; % factor de conversión de g a mmol
 
% Comidas (perturbaciones) a lo largo de un día
if t >= 0 && t < 180*60 % ingesta de 75 g de HC
    t1 = 0;
    Dg = 50*f;
end
 
% Ecuación
D = (Dg*Ag*(t-t1)*exp(-(t-t1)/Tmaxi))/(Vg*Tmaxg^2);

== matlab function MODELO_CORRECTO_BERGMAN_BASE/Ingesta 75 g7 ==
  data: in input; D output
function D = comida(in)
% Variables de entrada en la funcion
t = in(1) %- 8*60*60; % Ajuste para iniciar a las 8 de la mañana
 
% Parámetros del modelo
Ag = 0.8; % adimensional
Tmaxi = 55*60; % s
Vg = 13.79; % L
Tmaxg = 40*60; % s
t1 = 0;
Dg = 0;
f = 1000/180; % factor de conversión de g a mmol
 
% Comidas (perturbaciones) a lo largo de un día
if t >= 0 && t < 180*60 % ingesta de 75 g de HC
    t1 = 0;
    Dg = 50*f;
end
 
% Ecuación
D = (Dg*Ag*(t-t1)*exp(-(t-t1)/Tmaxi))/(Vg*Tmaxg^2);

== matlab function MODELO_CORRECTO_BERGMAN_BASE/Ingesta 75 g8 ==
  data: in input; D output
function D = comida(in)
% Variables de entrada en la funcion
t = in(1) %- 8*60*60; % Ajuste para iniciar a las 8 de la mañana
 
% Parámetros del modelo
Ag = 0.8; % adimensional
Tmaxi = 55*60; % s
Vg = 13.79; % L
Tmaxg = 40*60; % s
t1 = 0;
Dg = 0;
f = 1000/180; % factor de conversión de g a mmol
 
% Comidas (perturbaciones) a lo largo de un día
if t >= 0 && t < 180*60 % ingesta de 75 g de HC
    t1 = 0;
    Dg = 50*f;
end
 
% Ecuación
D = (Dg*Ag*(t-t1)*exp(-(t-t1)/Tmaxi))/(Vg*Tmaxg^2);

== matlab function MODELO_CORRECTO_BERGMAN_BASE/Ingesta 75 g10 ==
  data: in input; D output
function D = comida(in)
% Variables de entrada en la funcion
t = in(1) %- 8*60*60; % Ajuste para iniciar a las 8 de la mañana
 
% Parámetros del modelo
Ag = 0.8; % adimensional
Tmaxi = 55*60; % s
Vg = 13.79; % L
Tmaxg = 40*60; % s
t1 = 0;
Dg = 0;
f = 1000/180; % factor de conversión de g a mmol
 
% Comidas (perturbaciones) a lo largo de un día
if t >= 0 && t < 180*60 % ingesta de 75 g de HC
    t1 = 0;
    Dg = 50*f;
end
 
% Ecuación
D = (Dg*Ag*(t-t1)*exp(-(t-t1)/Tmaxi))/(Vg*Tmaxg^2);

== matlab function MODELO_CORRECTO_BERGMAN_BASE/Ingesta 75 g9 ==
  data: in input; D output
function D = comida(in)
% Variables de entrada en la funcion
t = in(1) %- 8*60*60; % Ajuste para iniciar a las 8 de la mañana
 
% Parámetros del modelo
Ag = 0.8; % adimensional
Tmaxi = 55*60; % s
Vg = 13.79; % L
Tmaxg = 40*60; % s
t1 = 0;
Dg = 0;
f = 1000/180; % factor de conversión de g a mmol
 
% Comidas (perturbaciones) a lo largo de un día
if t >= 0 && t < 180*60 % ingesta de 75 g de HC
    t1 = 0;
    Dg = 50*f;
end
 
% Ecuación
D = (Dg*Ag*(t-t1)*exp(-(t-t1)/Tmaxi))/(Vg*Tmaxg^2);

== matlab function MODELO_CORRECTO_BERGMAN_BASE/Ingesta 75 g11 ==
  data: in input; D output
function D = comida(in)
% Variables de entrada en la funcion
t = in(1) %- 8*60*60; % Ajuste para iniciar a las 8 de la mañana
 
% Parámetros del modelo
Ag = 0.8; % adimensional
Tmaxi = 55*60; % s
Vg = 13.79; % L
Tmaxg = 40*60; % s
t1 = 0;
Dg = 0;
f = 1000/180; % factor de conversión de g a mmol
 
% Comidas (perturbaciones) a lo largo de un día
if t >= 0 && t < 180*60 % ingesta de 75 g de HC
    t1 = 0;
    Dg = 50*f;
end
 
% Ecuación
D = (Dg*Ag*(t-t1)*exp(-(t-t1)/Tmaxi))/(Vg*Tmaxg^2);
